simulink model "controller13"  (R2023a)
settings: Solver=FixedStepAuto  StartTime=0.0  StopTime=mdl.exe_time  RelTol=1e-3
values from neighbouring files (symbols this model uses):
  ctr2 = ctr    [s1_setup.m]    (also in step1_setup.m)
  lut = gen_lut    [s1_setup.m]    (also in thrust2voltage_lut_20230809.mat = ; thrust2voltage_lut_20230829.mat = )
  mdl = make_model(mdl,rsim)    [s1_setup.m]    (also in setup_controller_with_functions.m = make_model(flight_time); step1_setup.m)
  use_simulation = 1    [step1_setup_v1.m]
undefined symbols (not defined in the file or in its folder): Angle, Axis, DiscIntNeverNeededParam, rjsim, servo_config, Standard_Devices, UDP_Protocol
libraries: simulink x25, sldrtlib x9, robotcorelib x8, dspmathops x3, dspswit3 x2, shared6dofsys x2, dspfdesign x2, sharedtransform x1, sharedutil x1, matrix_library x1, shared6dof x1, simulink_extras x1
(part 2 of 3)

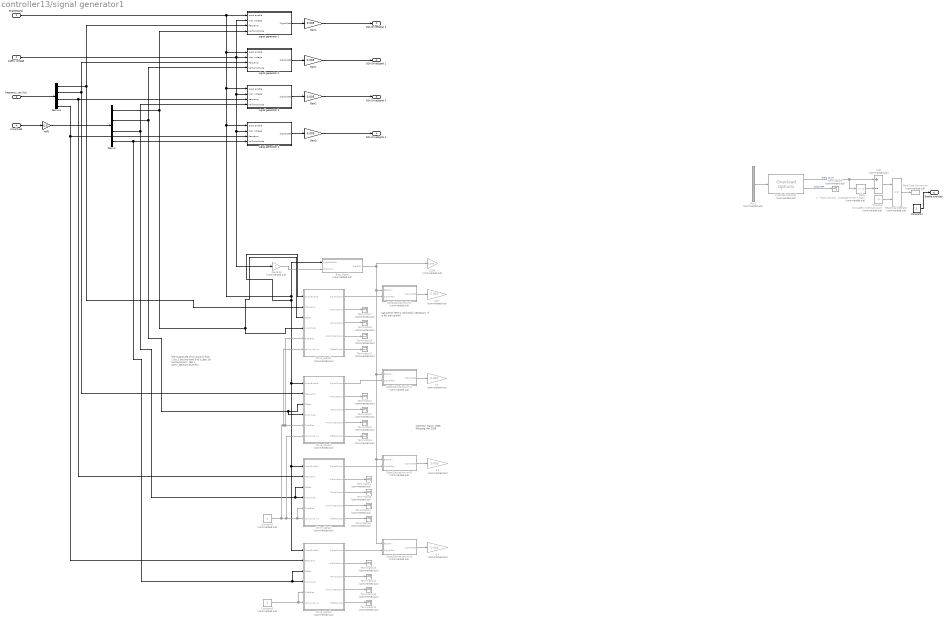
== system controller13/signal generator1 ==
  note: The magnitude of sin wave is from -1 to 1, but we want 0 to V_des. So we have 0.5*V_des + 0.5*V_des*sin(2*pi*f*t).
  note: Katie Byl
      | March, 2009
      |
      | Pakpong
      | Nov 2018
  note: saturation here is not totally necessary.
      | it is for pre-caution
  EnableSignal : Inport
  safety voltage : Inport  Port=2
  frequency_vec (hz) : Inport  Port=3
  Amplitude : Inport  Port=4
  0.2 : Gain  Commented=on  Gain=0.005
  0.3 : Gain  Commented=on  Gain=0.005
  0.4 : Gain  Commented=on  Gain=0.005
  1/200 : Gain  Commented=on  Gain=0.005
  Add : Sum  Commented=on  Inputs=+-
  Bias_Signal : Subsystem  Commented=on
  Constant : Constant  Commented=on  Value=ctr2.safety.overload.count
  Constant1 : Constant
  Constant2 : Constant  Commented=on  Value=0
  Constant3 : Constant  Commented=on  Value=0
  Data Type Conversion : DataTypeConversion  Commented=on  SaturateOnIntegerOverflow=off  RndMeth=Floor
  Delay : Delay  Commented=on  DelayLength=floor(ctr2.safety.overload.T*mdl.T_high)  InitialCondition=0
  Demux : Demux
  Demux1 : Demux
  Drive_Signal1 : Subsystem  Commented=on
  Drive_Signal2 : Subsystem  Commented=on
  Drive_Signal3 : Subsystem  Commented=on
  Drive_Signal4 : Subsystem  Commented=on
  Gain : Gain  Commented=on  Gain=0.005
  Gain{1..4} (4 alike) : Gain  Gain=0.005
  GainBias : Gain  Commented=on
  Mux2 : Mux  Commented=on
  Overload Options1 : slrealtimetgmanagement/Overload Options  Commented=on  startupDur=10  startupDurSrc=Tunable Parameter  maxOverload=1000  maxOverloadSrc=Tunable Parameter  TETFlag=on
  Relational Operator : RelationalOperator  Commented=on  Operator=<=  OutDataTypeStr=boolean  RndMeth=Simplest  InputSameDT=off
  SignalSaturationLimit : Subsystem  Commented=on
  SignalSaturationLimit1 : Subsystem  Commented=on
  SignalSaturationLimit2 : Subsystem  Commented=on
  SignalSaturationLimit3 : Subsystem  Commented=on
  Terminator{1..17} (17 alike) : Terminator  Commented=on
  half1 : Gain  Gain=0.5
  signal generator 1 : Subsystem
  signal generator 2 : Subsystem
  signal generator 3 : Subsystem
  signal generator 4 : Subsystem
  D2A DriveSignal 1 : Outport
  D2A DriveSignal 2 : Outport  Port=2
  D2A DriveSignal 3 : Outport  Port=3
  D2A DriveSignal 4 : Outport  Port=4
  Enable overload : Outport  Port=5
  wires:
  Bias_Signal/1(BiasD2A) -> 1/200/1, SignalSaturationLimit3/1(BiasMax), SignalSaturationLimit2/1(BiasMax), SignalSaturationLimit1/1(BiasMax), SignalSaturationLimit/1(BiasMax)
  EnableSignal/1 -> Drive_Signal1/1(QuasiEnable), Drive_Signal3/1(QuasiEnable), Drive_Signal2/1(QuasiEnable), Drive_Signal4/1(QuasiEnable), Bias_Signal/1(QuasiEnable), signal generator 4/1(quasi enable), signal generator 3/1(quasi enable), signal generator 2/1(quasi enable), signal generator 1/1(quasi enable)
  SignalSaturationLimit/1(SignalSatd) -> Gain/1
  GainBias/1 -> Bias_Signal/2(BiasVolts)
  SignalSaturationLimit1/1(SignalSatd) -> 0.2/1
  Amplitude/1 -> half1/1
  Drive_Signal3/4(AmplitudeOutput) -> Terminator15/1
  Drive_Signal3/2(WithoutRamp) -> Terminator13/1
  Drive_Signal3/3(RampOutput) -> Terminator14/1
  Drive_Signal3/5(OffsetOutput) -> Terminator12/1
  Drive_Signal2/3(RampOutput) -> Terminator8/1
  Drive_Signal2/4(AmplitudeOutput) -> Terminator11/1
  Drive_Signal3/1(SignalOutput) -> SignalSaturationLimit3/2(SignalRaw)
  Drive_Signal2/5(OffsetOutput) -> Terminator10/1
  Drive_Signal2/2(WithoutRamp) -> Terminator4/1
  Demux/3 -> Drive_Signal2/4(Amplitude), Drive_Signal2/3(Offset), signal generator 3/4(half amplitude)
  Demux/4 -> Drive_Signal3/4(Amplitude), Drive_Signal3/3(Offset), signal generator 4/4(half amplitude)
  Constant2/1 -> Drive_Signal1/6(split cycle mu), Drive_Signal1/5(PitchBias), Drive_Signal4/5(PitchBias), Drive_Signal4/6(split cycle mu), Drive_Signal2/5(PitchBias), Drive_Signal2/6(split cycle mu)
  Constant3/1 -> Drive_Signal3/5(PitchBias), Drive_Signal3/6(split cycle mu)
  SignalSaturationLimit2/1(SignalSatd) -> 0.3/1
  SignalSaturationLimit3/1(SignalSatd) -> 0.4/1
  Drive_Signal2/1(SignalOutput) -> SignalSaturationLimit2/2(SignalRaw)
  half1/1 -> Demux/1
  frequency_vec (hz)/1 -> Demux1/1
  Demux1/1 -> signal generator 1/3(frequency), Drive_Signal1/2(Frequency)
  Demux1/2 -> Drive_Signal4/2(Frequency), signal generator 2/3(frequency)
  Demux1/3 -> Drive_Signal2/2(Frequency), signal generator 3/3(frequency)
  Demux1/4 -> Drive_Signal3/2(Frequency), signal generator 4/3(frequency)
  Overload Options1/1 -> Delay/1, Add/1  "DrSig count"
  Overload Options1/2 -> Terminator3/1  "DrSig TET"
  Mux2/1 -> Overload Options1/1
  Delay/1 -> Add/2
  Add/1 -> Relational Operator/1
  Constant/1 -> Relational Operator/2
  Relational Operator/1 -> Data Type Conversion/1
  Drive_Signal4/1(SignalOutput) -> SignalSaturationLimit1/2(SignalRaw)
  Drive_Signal4/2(WithoutRamp) -> Terminator1/1
  Drive_Signal4/3(RampOutput) -> Terminator2/1
  Drive_Signal4/4(AmplitudeOutput) -> Terminator5/1
  Drive_Signal4/5(OffsetOutput) -> Terminator6/1
  Drive_Signal1/4(AmplitudeOutput) -> Terminator16/1
  Drive_Signal1/1(SignalOutput) -> SignalSaturationLimit/2(SignalRaw)
  Drive_Signal1/2(WithoutRamp) -> Terminator7/1
  Drive_Signal1/5(OffsetOutput) -> Terminator17/1
  Drive_Signal1/3(RampOutput) -> Terminator9/1
  Demux/1 -> Drive_Signal1/3(Offset), Drive_Signal1/4(Amplitude), signal generator 1/4(half amplitude)
  Constant1/1 -> Enable overload/1
  Demux/2 -> Drive_Signal4/4(Amplitude), Drive_Signal4/3(Offset), signal generator 2/4(half amplitude)
  safety voltage/1 -> GainBias/1, signal generator 4/2(max voltage), signal generator 3/2(max voltage), signal generator 1/2(max voltage), signal generator 2/2(max voltage)
  signal generator 2/1(SignalSatd) -> Gain1/1
  signal generator 3/1(SignalSatd) -> Gain2/1
  signal generator 4/1(SignalSatd) -> Gain3/1
  signal generator 1/1(SignalSatd) -> Gain4/1
  Gain3/1 -> D2A DriveSignal 4/1
  Gain2/1 -> D2A DriveSignal 3/1
  Gain1/1 -> D2A DriveSignal 2/1
  Gain4/1 -> D2A DriveSignal 1/1

== system controller13/signal safety (no imag & NaN) ==
  In1 : Inport
  Complex to Real-Imag{,1..3} (4 alike) : ComplexToRealImag
  Constant{,1..3} (4 alike) : Constant  Value=0
  Demux : Demux
  IsNaN{,1..3} (4 alike) : RelationalOperator  Operator=isNaN  OutDataTypeStr=boolean  RndMeth=Simplest  InputSameDT=off
  Mux : Mux
  Switch{1..3,17} (4 alike) : Switch  Criteria=u2 > Threshold  SaturateOnIntegerOverflow=off  InputSameDT=off
  Terminator{,1..3} (4 alike) : Terminator
  Output : Outport
  wires:
  In1/1 -> Demux/1
  IsNaN/1 -> Switch17/2
  Constant/1 -> Switch17/1
  Switch17/1 -> Complex to Real-Imag/1
  Complex to Real-Imag/2 -> Terminator/1
  Demux/1 -> Switch17/3, IsNaN/1
  Complex to Real-Imag1/2 -> Terminator1/1
  Complex to Real-Imag1/1 -> Mux/2
  IsNaN1/1 -> Switch1/2
  Switch1/1 -> Complex to Real-Imag1/1
  Demux/2 -> Switch1/3, IsNaN1/1
  Constant1/1 -> Switch1/1
  Complex to Real-Imag2/2 -> Terminator2/1
  Complex to Real-Imag2/1 -> Mux/3
  IsNaN2/1 -> Switch2/2
  Switch2/1 -> Complex to Real-Imag2/1
  Demux/3 -> Switch2/3, IsNaN2/1
  Constant2/1 -> Switch2/1
  Complex to Real-Imag3/2 -> Terminator3/1
  Complex to Real-Imag3/1 -> Mux/4
  IsNaN3/1 -> Switch3/2
  Demux/4 -> IsNaN3/1, Switch3/3
  Switch3/1 -> Complex to Real-Imag3/1
  Constant3/1 -> Switch3/1
  Mux/1 -> Output/1
  Complex to Real-Imag/1 -> Mux/1

== system controller13/stance climbing subsystem ==
  Action Port : ActionPort  ActionPortLabel=default:
  Constant7 : Constant  Value=[0;0;1]
  Out1 : Outport
  wires:
  Constant7/1 -> Out1/1

== system controller13/sync with Speedgoat ==
  Gain3 : Gain  OutDataTypeStr=uint8
  Packet Output2 : sldrtlib/Packet Output  SampleTime=1/2000  MaxMissedTicks=100  ShowMissedTicks=off  YieldWhenWaiting=off  DrvName=Standard_Devices/UDP_Protocol  DrvAddress=16300  DrvOptions=[0 24000 49 54 57 46 50 53 52 46 49 48 51 46 52 48 0 0 0 0 0 0 0 0 0 0 0 0 0 0 0 0 0 0 0 0 0 0 0 0 0 0 0 0 0 0 0 0 0 0 0 0 0 0 0 0 0 0 0 0 0 0 0 0 0 0 0 0 0 0 0 0 0 0 0 0 0 0 0 0 0 0 0 0 0 0 0 0 0 0 0 0 0 0 0 0 0 0 0 0 0 0 0 0 0 0 0 0 0 0 0 0 0 0 0 0 0 0 0 0 0 0 0 0 0 0 0 0 0 0 0 0 0 0 0 0 0 0 0 0 0 0 0 0 0 0 0 0 0 0 0 0 0 0 0 0 0 0 0 0 0 0 0 0 0 0 0 0 0 0 0 0 0 0 0 0 0 0 0 0 0 0 0 0 0 0 0 0 0 0 0 0 0 0 0 0 0 0 0 0 0 0 0 0 0 0 0 0 0 0 0 0 0 0 0 0 0 0 0 0 0 0 0 0 0 0 0 0 0 0 0 0 0 0 0 0 0 0 0 0 0 0 0 0 0 0 0 0 0 0 0 0 0 0 0 0]  PacketSize=1  DataTypes='1*uint8'  ShowReady=off  ShowError=off  PacketID=1  ByteOrder=1  InitialValue=[]  FinalValue=[]
      settings: AttributesFormatString=UDP Protocol [16300]
  Pulse Generator : DiscretePulseGenerator  Period=1000  PulseWidth=500  SampleTime=1/2000
  Scope : Scope
  wires:
  Pulse Generator/1 -> Gain3/1
  Gain3/1 -> Packet Output2/1, Scope/1

== system controller13/voltage safety (no imag & NaN) ==
  In1 : Inport
  Complex to Real-Imag{,1..3} (4 alike) : ComplexToRealImag
  Delay{,1..3} (4 alike) : Delay  DelayLength=1
  Demux : Demux
  IsNaN{,1..3} (4 alike) : RelationalOperator  Operator=isNaN  OutDataTypeStr=boolean  RndMeth=Simplest  InputSameDT=off
  Mux : Mux
  Switch{1..3,17} (4 alike) : Switch  Criteria=u2 > Threshold  SaturateOnIntegerOverflow=off  InputSameDT=off
  Terminator{,1..3} (4 alike) : Terminator
  Output : Outport
  wires:
  In1/1 -> Demux/1
  IsNaN/1 -> Switch17/2
  Switch17/1 -> Delay1/1, Complex to Real-Imag/1
  Complex to Real-Imag/2 -> Terminator/1
  Demux/1 -> Switch17/3, IsNaN/1
  Complex to Real-Imag1/2 -> Terminator1/1
  Complex to Real-Imag1/1 -> Mux/2
  IsNaN1/1 -> Switch1/2
  Switch1/1 -> Delay/1, Complex to Real-Imag1/1
  Demux/2 -> Switch1/3, IsNaN1/1
  Complex to Real-Imag2/2 -> Terminator2/1
  Complex to Real-Imag2/1 -> Mux/3
  IsNaN2/1 -> Switch2/2
  Switch2/1 -> Delay2/1, Complex to Real-Imag2/1
  Demux/3 -> Switch2/3, IsNaN2/1
  Complex to Real-Imag3/2 -> Terminator3/1
  Complex to Real-Imag3/1 -> Mux/4
  IsNaN3/1 -> Switch3/2
  Demux/4 -> IsNaN3/1, Switch3/3
  Switch3/1 -> Delay3/1, Complex to Real-Imag3/1
  Mux/1 -> Output/1
  Complex to Real-Imag/1 -> Mux/1
  Delay/1 -> Switch1/1
  Delay1/1 -> Switch17/1
  Delay2/1 -> Switch2/1
  Delay3/1 -> Switch3/1

== system controller13/yaw-free attitude controller ==
  desired_z_b : Inport
  R : Inport  Port=2
  omega_b : Inport  Port=3
  Add1 : Sum  Inputs=-+|
  Constant4 : Constant  Value=[0;0;1]
  Cross Product : vrlib/Utilities/Cross Product
  Gain : Gain  Gain=-1
  Matrix Multiply2 : Product  Multiplication=Matrix(*)
  Matrix Multiply5 : Product  Multiplication=Matrix(*)
  Product1 : Product
  Product2 : Product
  Transpose : Math  Operator=transpose
  d_gain : Constant  Value=[30;37;0]
  p_gain : Constant  Value=[350;600;0]
  z_b : Outport
  torque_b : Outport  Port=2
  wires:
  d_gain/1 -> Product1/2
  desired_z_b/1 -> Cross Product/1
  Constant4/1 -> Matrix Multiply2/2
  Matrix Multiply2/1 -> z_b/1, Cross Product/2
  R/1 -> Matrix Multiply2/1, Transpose/1
  Gain/1 -> Matrix Multiply5/2
  Cross Product/1 -> Gain/1
  Product1/1 -> Add1/1
  Add1/1 -> torque_b/1
  omega_b/1 -> Product1/1
  Transpose/1 -> Matrix Multiply5/1  "R^T"
  Matrix Multiply5/1 -> Product2/1
  p_gain/1 -> Product2/2
  Product2/1 -> Add1/2

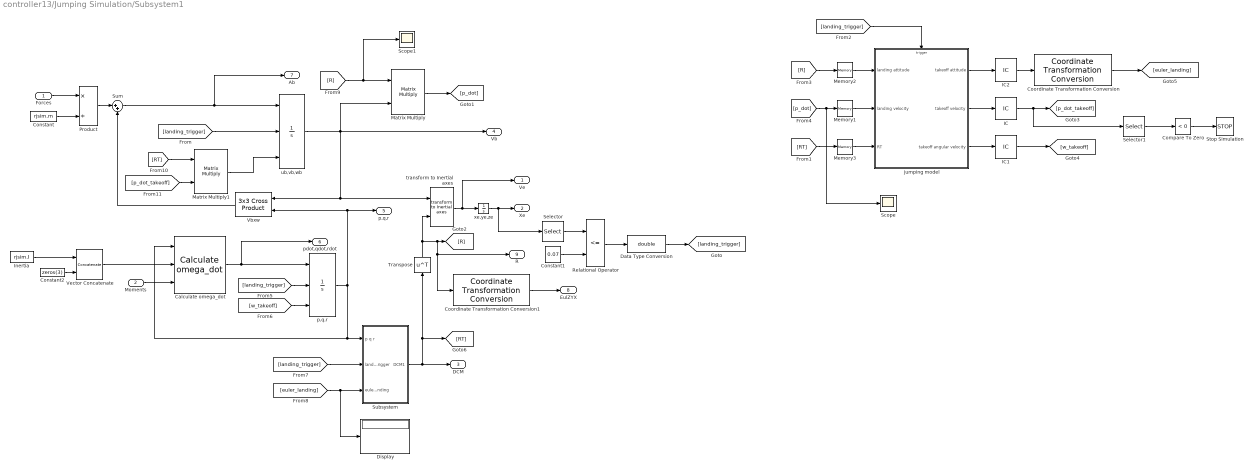
== system controller13/Jumping Simulation/Subsystem1 ==
  Forces : Inport  OutDataTypeStr=double  Unit=N  PortDimensions=3
  Moments : Inport  Port=2  OutDataTypeStr=double  Unit=N*m  PortDimensions=3
  Calculate omega_dot : shared6dofsys/Calculate omega_dot  aMode=aMode
  Compare To Zero : simulink/Logic and Bit Operations/Compare To Zero  relop=<  OutDataTypeStr=boolean
  Constant : Constant  Value=rjsim.m  OutDataTypeStr=Inherit: Inherit via back propagation
  Constant1 : Constant  Value=0.07
  Constant2 : Constant  Value=zeros(3)
  Coordinate Transformation Conversion : robotcorelib/Coordinate Transformation Conversion  InputRepresentation=Rotation Matrix  InputEulerSequence=ZYX  ShowTrVecInputPort=on  OutputRepresentation=Euler Angles  OutputEulerSequence=ZYX  ShowTrVecOutputPort=on  SimulateUsing=Interpreted execution
      settings: LibrarySourceBlock=navlib/Utilities/Coordinate Transformation Conversion
  Coordinate Transformation Conversion1 : robotcorelib/Coordinate Transformation Conversion  InputRepresentation=Rotation Matrix  InputEulerSequence=ZYX  ShowTrVecInputPort=on  OutputRepresentation=Euler Angles  OutputEulerSequence=ZYX  ShowTrVecOutputPort=on  SimulateUsing=Interpreted execution
      settings: LibrarySourceBlock=navlib/Utilities/Coordinate Transformation Conversion
  Data Type Conversion : DataTypeConversion  OutDataTypeStr=double  SaturateOnIntegerOverflow=off  RndMeth=Floor
  Display : Display
  IC : InitialCondition  Value=rjsim.v0
  IC1 : InitialCondition  Value=[0,0,0]
  IC2 : InitialCondition  Value=rjsim.rotm0
  Inertia : Constant  Value=rjsim.I  OutDataTypeStr=Inherit: Inherit via back propagation
  Matrix Multiply : Product  Multiplication=Matrix(*)
  Matrix Multiply1 : Product  Multiplication=Matrix(*)
  Memory1 : Memory
  Memory2 : Memory
  Memory3 : Memory
  Product : Product  Inputs=*/  SaturateOnIntegerOverflow=on  OutDataTypeStr=Inherit: Same as first input
  Relational Operator : RelationalOperator  Operator=<=  OutDataTypeStr=boolean  RndMeth=Simplest  InputSameDT=off
  Scope : Scope
  Scope1 : Scope
  Selector : Selector  InputPortWidth=3  IndexOptions=Index vector (dialog)  Indices=[3]  OutputSizes=1
  Selector1 : Selector  InputPortWidth=3  IndexOptions=Index vector (dialog)  Indices=[3]  OutputSizes=1
  Stop Simulation : Stop
  Subsystem : Subsystem
  Sum : Sum  Inputs=|++  SaturateOnIntegerOverflow=on
  Transpose : Math  Operator=transpose  SignedPower=on
  Vbxw : sharedutil/3x3 Cross Product  aMode=aMode
  Vector Concatenate : Concatenate  Mode=Multidimensional array
  jumping model : Subsystem  TreatAsAtomicUnit=on
  "p,q,r " : Integrator  ExternalReset=rising  InitialConditionSource=external  InitialCondition=[0,0,0]
  "transform to Inertial axes " : shared6dof/6DOF (Euler Angles)/transform to Inertial axes   SystemSampleTime=-1  VariantActivationTime=update diagram  Latency=0  AutoFrameSizeCalculation=off
  ub,vb,wb : Integrator  ExternalReset=rising  InitialConditionSource=external  InitialCondition=[0,0,0]
  xe,ye,ze : Integrator  InitialCondition=rjsim.p0
  Ve : Outport  OutDataTypeStr=double  Unit=m/s  VectorParamsAs1DForOutWhenUnconnected=off
  Xe : Outport  Port=2  OutDataTypeStr=double  Unit=m  VectorParamsAs1DForOutWhenUnconnected=off
  DCM : Outport  Port=3  OutDataTypeStr=double  Unit=1  VectorParamsAs1DForOutWhenUnconnected=off
  Vb : Outport  Port=4  OutDataTypeStr=double  Unit=m/s  VectorParamsAs1DForOutWhenUnconnected=off
  p,q,r : Outport  Port=5  OutDataTypeStr=double  Unit=rad/s  VectorParamsAs1DForOutWhenUnconnected=off
  pdot,qdot,rdot : Outport  Port=6  OutDataTypeStr=double  Unit=rad/s^2  VectorParamsAs1DForOutWhenUnconnected=off
  Ab : Outport  Port=7  OutDataTypeStr=double  Unit=m/s^2  VectorParamsAs1DForOutWhenUnconnected=off
  EulZYX : Outport  Port=8
  R : Outport  Port=9
  wires:
  "transform to Inertial axes "/1 -> Ve/1, xe,ye,ze/1
  Constant/1 -> Product/2
  Product/1 -> Sum/1
  xe,ye,ze/1 -> Selector/1, Xe/1
  ub,vb,wb/1 -> Vb/1, Matrix Multiply/2, Vbxw/1, "transform to Inertial axes "/1
  Sum/1 -> Ab/1, ub,vb,wb/1
  Vbxw/1 -> Sum/2
  "p,q,r "/1 -> Calculate omega_dot/1, Subsystem/1("p q r "), Vbxw/2, p,q,r/1
  Subsystem/1(DCM1) -> Transpose/1, [RT], DCM/1
  Forces/1 -> Product/1
  Transpose/1 -> Coordinate Transformation Conversion1/1, R/1, [R], "transform to Inertial axes "/2
  Calculate omega_dot/1 -> pdot,qdot,rdot/1, "p,q,r "/1
  Moments/1 -> Calculate omega_dot/3
  Vector Concatenate/1 -> Calculate omega_dot/2
  Constant2/1 -> Vector Concatenate/2
  Inertia/1 -> Vector Concatenate/1
  Constant1/1 -> Relational Operator/2
  Selector/1 -> Relational Operator/1
  Relational Operator/1 -> Data Type Conversion/1
  [landing_trigger] -> ub,vb,wb/2
  [landing_trigger] -> jumping model/Trigger
  [R] -> Memory2/1
  [p_dot] -> Scope/1, Memory1/1
  Memory1/1 -> jumping model/2(landing velocity)
  Memory2/1 -> jumping model/1(landing attitude)
  jumping model/2(takeoff velocity) -> IC/1
  [landing_trigger] -> "p,q,r "/2
  jumping model/3(takeoff angular velocity) -> IC1/1
  [w_takeoff] -> "p,q,r "/3
  [landing_trigger] -> Subsystem/2(landing trigger)
  jumping model/1(takeoff attitude) -> IC2/1
  Coordinate Transformation Conversion/1 -> [euler_landing]
  Data Type Conversion/1 -> [landing_trigger]
  IC/1 -> Selector1/1, [p_dot_takeoff]
  IC1/1 -> [w_takeoff]
  IC2/1 -> Coordinate Transformation Conversion/1
  [R] -> Scope1/1, Matrix Multiply/1
  Matrix Multiply/1 -> [p_dot]
  [RT] -> Matrix Multiply1/1
  [p_dot_takeoff] -> Matrix Multiply1/2
  Matrix Multiply1/1 -> ub,vb,wb/3
  Coordinate Transformation Conversion1/1 -> EulZYX/1
  [RT] -> Memory3/1
  Memory3/1 -> jumping model/3(RT)
  Selector1/1 -> Compare To Zero/1
  Compare To Zero/1 -> Stop Simulation/1
  [euler_landing] -> Display/1, Subsystem/3(euler_landing)

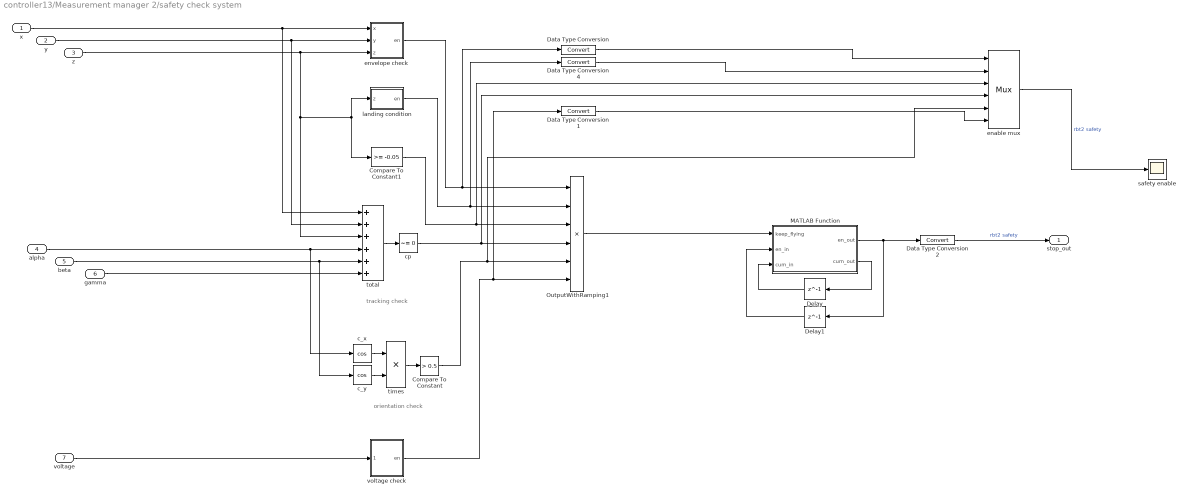
== system controller13/Measurement manager 2/safety check system ==
  note: orientation check
  note: tracking check
  x : Inport
  y : Inport  Port=2
  z : Inport  Port=3
  alpha : Inport  Port=4
  beta : Inport  Port=5
  gamma : Inport  Port=6
  voltage : Inport  Port=7
  Compare To Constant : simulink/Logic and Bit Operations/Compare To Constant  relop=>  const=0.5  OutDataTypeStr=uint8
  Compare To Constant1 : simulink/Logic and Bit Operations/Compare To Constant  relop=>=  const=-0.05  OutDataTypeStr=uint8
  Data Type Conversion{,1..2,4} (4 alike) : DataTypeConversion  SaturateOnIntegerOverflow=off  RndMeth=Floor
  Delay : Delay  DelayLength=1
  Delay1 : Delay  DelayLength=1  InitialCondition=1
  MATLAB Function : MATLAB Function  TreatAsAtomicUnit=on
  OutputWithRamping1 : Product  Inputs=6  RndMeth=Zero
  c_x : Trigonometry  Operator=cos
  c_y : Trigonometry  Operator=cos
  cp : simulink/Logic and Bit Operations/Compare To Zero  relop=~=  OutDataTypeStr=uint8
  enable mux : Mux  Inputs=6
      settings: DisplayOption=signals
  envelope check : MATLAB Function  TreatAsAtomicUnit=on
  landing condition : Subsystem
  safety enable : Scope
  times : Product  RndMeth=Zero
  total : Sum  Inputs=++++++
  voltage check : MATLAB Function  TreatAsAtomicUnit=on  SystemSampleTime=mdl.T
  stop_out : Outport
  wires:
  Compare To Constant1/1 -> enable mux/3, OutputWithRamping1/3
  y/1 -> envelope check/2(y), total/2
  cp/1 -> enable mux/4, OutputWithRamping1/4
  envelope check/1(en) -> Data Type Conversion/1, OutputWithRamping1/1
  enable mux/1 -> safety enable/1  "rbt2 safety"
  landing condition/1(en) -> Data Type Conversion4/1, OutputWithRamping1/2
  Data Type Conversion/1 -> enable mux/1
  times/1 -> Compare To Constant/1
  voltage check/1(en) -> Data Type Conversion1/1, OutputWithRamping1/6
  z/1 -> total/3, Compare To Constant1/1, landing condition/1(z), envelope check/3(z)
  Compare To Constant/1 -> enable mux/5, OutputWithRamping1/5
  total/1 -> cp/1
  Data Type Conversion4/1 -> enable mux/2
  x/1 -> total/1, envelope check/1(x)
  alpha/1 -> total/4, c_x/1
  beta/1 -> total/5, c_y/1
  c_x/1 -> times/1
  c_y/1 -> times/2
  Data Type Conversion1/1 -> enable mux/6
  voltage/1 -> voltage check/1(voltage)
  gamma/1 -> total/6
  OutputWithRamping1/1 -> MATLAB Function/1(keep_flying)
  Delay1/1 -> MATLAB Function/2(en_in)
  MATLAB Function/1(en_out) -> Delay1/1, Data Type Conversion2/1
  Delay/1 -> MATLAB Function/3(cum_in)
  MATLAB Function/2(cum_out) -> Delay/1
  Data Type Conversion2/1 -> stop_out/1  "rbt2 safety"

== system controller13/Subsystem6/Subsystem4 ==
  In1 : Inport
  data ready : Inport  Port=2
  Add1 : Sum  Inputs=+-
  Add2 : Sum  Inputs=+-
  Digital Clock : DigitalClock  SampleTime=1/10000
  If : If  IfExpression=u1 == 0
  If Action Subsystem : Subsystem  TreatAsAtomicUnit=on
  If Action Subsystem1 : Subsystem  TreatAsAtomicUnit=on
  Merge : Merge
  Triggered Subsystem : Subsystem  TreatAsAtomicUnit=on
  p dot : Outport
  wires:
  In1/1 -> Triggered Subsystem/1(In1)
  data ready/1 -> Triggered Subsystem/Trigger
  Triggered Subsystem/1(Out1) -> Add1/1
  Triggered Subsystem/2(Output) -> Add1/2
  Triggered Subsystem/3(Output1) -> Add2/1
  Triggered Subsystem/4(Output2) -> Add2/2
  Add1/1 -> If Action Subsystem/1(In1)
  Add2/1 -> If Action Subsystem/2(In2), If/1
  If/2 -> If Action Subsystem/Action
  If/1 -> If Action Subsystem1/Action
  If Action Subsystem1/1(Out1) -> Merge/2
  If Action Subsystem/1(Out1) -> Merge/1
  Merge/1 -> p dot/1
  Digital Clock/1 -> Triggered Subsystem/2(In2)

== system controller13/Subsystem6/Subsystem5 ==
  euler_angles : Inport
  data ready : Inport  Port=2
  sim enable : Inport  Port=3
  Add1 : Sum  Inputs=+-
  Add2 : Sum  Inputs=+-
  Add3 : Sum  Inputs=+-
  Delay : Delay  DelayLength=25  InitialCondition=zeros(9,25)
  Digital Clock : DigitalClock  SampleTime=1/10000
  Gain : Gain  Gain=1/(25/10000)
  If : If  IfExpression=u1 == 0
  If Action Subsystem : Subsystem  TreatAsAtomicUnit=on
  If Action Subsystem1 : Subsystem  TreatAsAtomicUnit=on
  Merge : Merge
  Rotation Matrix : MATLAB Function  TreatAsAtomicUnit=on
  Rotation Matrix1 : MATLAB Function  TreatAsAtomicUnit=on
  Switch1 : Switch  Criteria=u2 > Threshold  SaturateOnIntegerOverflow=off  InputSameDT=off
  Triggered Subsystem : Subsystem  TreatAsAtomicUnit=on
  R : Outport
  Rdot : Outport  Port=2
  Omega : Outport  Port=3
  wires:
  Triggered Subsystem/1(Out1) -> Add1/1
  Triggered Subsystem/3(Output1) -> Add2/1
  Triggered Subsystem/4(Output2) -> Add2/2
  If Action Subsystem1/1(Out1) -> Merge/2
  If Action Subsystem/1(Out1) -> Merge/1
  Triggered Subsystem/2(Output) -> Add1/2
  Digital Clock/1 -> Triggered Subsystem/2(In2)
  data ready/1 -> Triggered Subsystem/Trigger
  Add2/1 -> If Action Subsystem/2(In2), If/1
  If/2 -> If Action Subsystem/Action
  If/1 -> If Action Subsystem1/Action
  Add1/1 -> If Action Subsystem/1(In1)
  euler_angles/1 -> Rotation Matrix/1(euler_angles)
  Rotation Matrix/1(R) -> Triggered Subsystem/1(R), Delay/1, Add3/1, R/1, Rotation Matrix1/1(R)
  Rotation Matrix1/1(w) -> Omega/1  "p_filt"
  Delay/1 -> Add3/2
  Add3/1 -> Gain/1
  Gain/1 -> Switch1/1
  sim enable/1 -> Switch1/2
  Merge/1 -> Switch1/3
  Switch1/1 -> Rotation Matrix1/2(Rdot), Rdot/1  "p_raw"

== system controller13/UDP send to Arduino/HV amplifier gains ==
  high voltage 1 : Inport
  high voltage 2 : Inport  Port=2
  high voltage 3 : Inport  Port=3
  high voltage 4 : Inport  Port=4
  Gain{4..7} (4 alike) : Gain
  DAC voltage 1 : Outport
  DAC voltage 2 : Outport  Port=2
  DAC voltage 3 : Outport  Port=3
  DAC voltage 4 : Outport  Port=4
  wires:
  Gain5/1 -> DAC voltage 2/1  "DAC voltage 2"
  Gain4/1 -> DAC voltage 1/1  "DAC voltage 1"
  high voltage 2/1 -> Gain5/1
  Gain7/1 -> DAC voltage 4/1  "DAC voltage 4"
  high voltage 1/1 -> Gain4/1
  Gain6/1 -> DAC voltage 3/1  "DAC voltage 3"
  high voltage 3/1 -> Gain6/1
  high voltage 4/1 -> Gain7/1

== system controller13/UDP send to Arduino/UDP send to Arduino DAC ==
  note: Aptinex DAC 20230818
  DAC1 : Inport
  DAC2 : Inport  Port=2
  DAC3 : Inport  Port=3
  DAC4 : Inport  Port=4
  DO2 : Inport  Port=5  OutDataTypeStr=boolean
  Bit Set : simulink/Logic and Bit Operations/Bit Set  iBit=12
  Demux : Demux
  Gain : Gain  Gain=4095/10.28  OutDataTypeStr=uint16
  Gain1 : Gain  Gain=4095/10.68  OutDataTypeStr=uint16
  Gain2 : Gain  Gain=4095/10.44  OutDataTypeStr=uint16
  Gain3 : Gain  Gain=4095/10  OutDataTypeStr=uint16
  Mux : Mux
  Mux1 : Mux
  Saturation : Saturate  UpperLimit=10  LowerLimit=0
  Switch : Switch  Criteria=u2 ~= 0  OutDataTypeStr=uint16  SaturateOnIntegerOverflow=off  InputSameDT=off
  Output : Outport
  wires:
  Gain3/1 -> Mux1/4  "UDP uint16 4"
  Gain1/1 -> Mux1/2  "UDP uint16 2"
  Gain/1 -> Bit Set/1, Switch/3  "UDP uint16 1"
  Gain2/1 -> Mux1/3  "UDP uint16 3"
  DO2/1 -> Switch/2
  Bit Set/1 -> Switch/1
  Mux1/1 -> Output/1
  Switch/1 -> Mux1/1
  Demux/1 -> Gain/1
  Demux/2 -> Gain1/1
  Demux/3 -> Gain2/1
  Demux/4 -> Gain3/1
  DAC1/1 -> Mux/1  "DAC voltage 1"
  DAC2/1 -> Mux/2  "DAC voltage 2"
  DAC3/1 -> Mux/3  "DAC voltage 3"
  DAC4/1 -> Mux/4  "DAC voltage 4"
  Mux/1 -> Saturation/1
  Saturation/1 -> Demux/1

== system controller13/get xy ini/Subsystem ==
  In1 : Inport
  Trigger : TriggerPort  VariantControl=Variant  PortDimensions=1
  Out1 : Outport
  wires:
  In1/1 -> Out1/1

== system controller13/servo control/servowrite ==
  In1 : Inport
  Add : Sum  Inputs=|+-
  Add1 : Sum  Inputs=|+-
  Add2 : Sum  Inputs=|+-
  Constant2 : Constant  Value=700
  Constant3 : Constant  Value=90
  Constant4 : Constant  Value=-1500
  Data Type Conversion : DataTypeConversion  OutDataTypeStr=uint16  SaturateOnIntegerOverflow=off  RndMeth=Floor
  Gain : Gain  Gain=800/76
  Packet Output : sldrtlib/Packet Output  SampleTime=1/400  MaxMissedTicks=100  ShowMissedTicks=off  YieldWhenWaiting=off  DrvName=Standard_Devices/UDP_Protocol  DrvAddress=25005  DrvOptions=[0 25000 49 54 57 46 50 53 52 46 49 48 51 46 52 57 0 0 0 0 0 0 0 0 0 0 0 0 0 0 0 0 0 0 0 0 0 0 0 0 0 0 0 0 0 0 0 0 0 0 0 0 0 0 0 0 0 0 0 0 0 0 0 0 0 0 0 0 0 0 0 0 0 0 0 0 0 0 0 0 0 0 0 0 0 0 0 0 0 0 0 0 0 0 0 0 0 0 0 0 0 0 0 0 0 0 0 0 0 0 0 0 0 0 0 0 0 0 0 0 0 0 0 0 0 0 0 0 0 0 0 0 0 0 0 0 0 0 0 0 0 0 0 0 0 0 0 0 0 0 0 0 0 0 0 0 0 0 0 0 0 0 0 0 0 0 0 0 0 0 0 0 0 0 0 0 0 0 0 0 0 0 0 0 0 0 0 0 0 0 0 0 0 0 0 0 0 0 0 0 0 0 0 0 0 0 0 0 0 0 0 0 0 0 0 0 0 0 0 0 0 0 0 0 0 0 0 0 0 0 0 0 0 0 0 0 0 0 0 0 0 0 0 0 0 0 0 0 0 0 0 0 0 0 0 0]  PacketSize=2  DataTypes='1*uint16'  ShowReady=off  ShowError=off  PacketID=1  ByteOrder=1  InitialValue=[]  FinalValue=[]
      settings: AttributesFormatString=UDP Protocol [25005]
  Saturation : Saturate  UpperLimit=2300  LowerLimit=700
  wires:
  Add2/1 -> Saturation/1
  Data Type Conversion/1 -> Packet Output/1
  Constant2/1 -> Add/2
  Constant4/1 -> Add2/2
  Gain/1 -> Add2/1
  Add/1 -> Data Type Conversion/1
  In1/1 -> Add1/1
  Saturation/1 -> Add/1
  Constant3/1 -> Add1/2
  Add1/1 -> Gain/1

== system controller13/signal generator1/Bias_Signal ==
  note: time constant = 0.002sec
  QuasiEnable : Inport
  BiasVolts : Inport  Port=2
  AveragedBias : Subsystem
  PreGain : Gain
  Product : Product  RndMeth=Zero
  SIgnalForRamp_binary : Subsystem
  SaturatingRamp : DiscreteIntegrator  gainval=100  SampleTime=-1  LimitOutput=on  UpperSaturationLimit=1  LowerSaturationLimit=0  ICPrevOutput=DiscIntNeverNeededParam  ICPrevScaledInput=DiscIntNeverNeededParam
  BiasD2A : Outport
  wires:
  PreGain/1 -> BiasD2A/1
  BiasVolts/1 -> AveragedBias/1(In1)
  QuasiEnable/1 -> SIgnalForRamp_binary/1(In1)
  SIgnalForRamp_binary/1(Out1) -> SaturatingRamp/1
  SaturatingRamp/1 -> Product/1
  AveragedBias/1(Out1) -> Product/2
  Product/1 -> PreGain/1

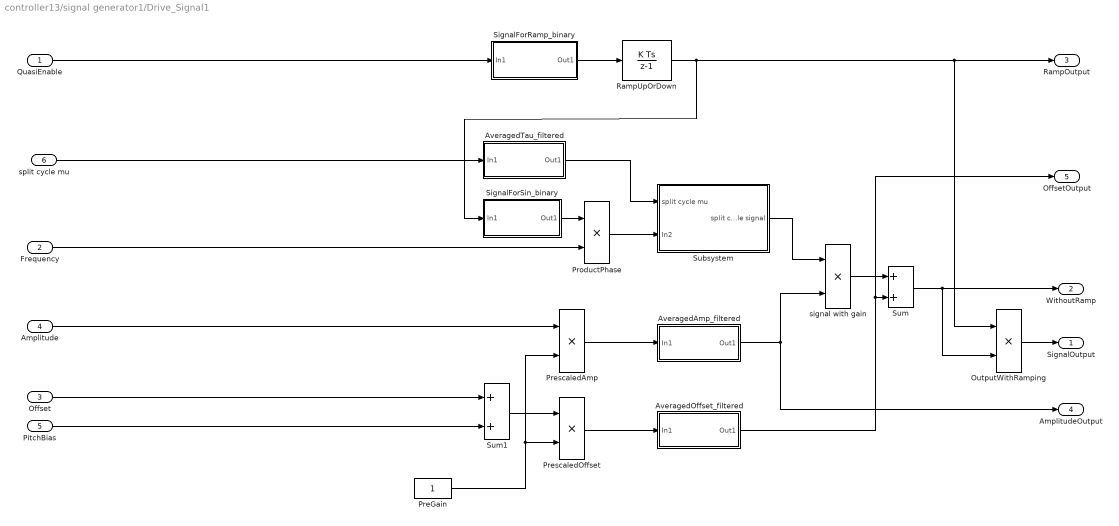
== system controller13/signal generator1/Drive_Signal1 ==
  QuasiEnable : Inport
  Frequency : Inport  Port=2
  Offset : Inport  Port=3
  Amplitude : Inport  Port=4
  PitchBias : Inport  Port=5
  split cycle mu : Inport  Port=6
  AveragedAmp_filtered : Subsystem
  AveragedOffset_filtered : Subsystem
  AveragedTau_filtered : Subsystem
  OutputWithRamping : Product  RndMeth=Zero
  PreGain : Constant
  PrescaledAmp : Product  RndMeth=Zero
  PrescaledOffset : Product  RndMeth=Zero
  ProductPhase : Product  RndMeth=Zero
  RampUpOrDown : DiscreteIntegrator  gainval=100  SampleTime=-1  LimitOutput=on  UpperSaturationLimit=1  LowerSaturationLimit=0  ICPrevOutput=DiscIntNeverNeededParam  ICPrevScaledInput=DiscIntNeverNeededParam
  SignalForRamp_binary : Subsystem
  SignalForSin_binary : Subsystem
  Subsystem : Subsystem
  Sum : Sum
  Sum1 : Sum
  signal with gain : Product  RndMeth=Zero
  SignalOutput : Outport
  WithoutRamp : Outport  Port=2
  RampOutput : Outport  Port=3
  AmplitudeOutput : Outport  Port=4
  OffsetOutput : Outport  Port=5
  wires:
  PrescaledAmp/1 -> AveragedAmp_filtered/1(In1)
  Sum/1 -> OutputWithRamping/2, WithoutRamp/1
  RampUpOrDown/1 -> RampOutput/1, OutputWithRamping/1, SignalForSin_binary/1(In1)
  QuasiEnable/1 -> SignalForRamp_binary/1(In1)
  SignalForRamp_binary/1(Out1) -> RampUpOrDown/1
  Amplitude/1 -> PrescaledAmp/1
  signal with gain/1 -> Sum/1
  Frequency/1 -> ProductPhase/2
  SignalForSin_binary/1(Out1) -> ProductPhase/1
  ProductPhase/1 -> Subsystem/2(In2)
  AveragedOffset_filtered/1(Out1) -> Sum/2, OffsetOutput/1
  PrescaledOffset/1 -> AveragedOffset_filtered/1(In1)
  PreGain/1 -> PrescaledAmp/2, PrescaledOffset/2
  OutputWithRamping/1 -> SignalOutput/1
  AveragedAmp_filtered/1(Out1) -> signal with gain/2, AmplitudeOutput/1
  Sum1/1 -> PrescaledOffset/1
  Offset/1 -> Sum1/1
  PitchBias/1 -> Sum1/2
  AveragedTau_filtered/1(Out1) -> Subsystem/1(split cycle mu)
  split cycle mu/1 -> AveragedTau_filtered/1(In1)
  Subsystem/1(split cycle signal) -> signal with gain/1

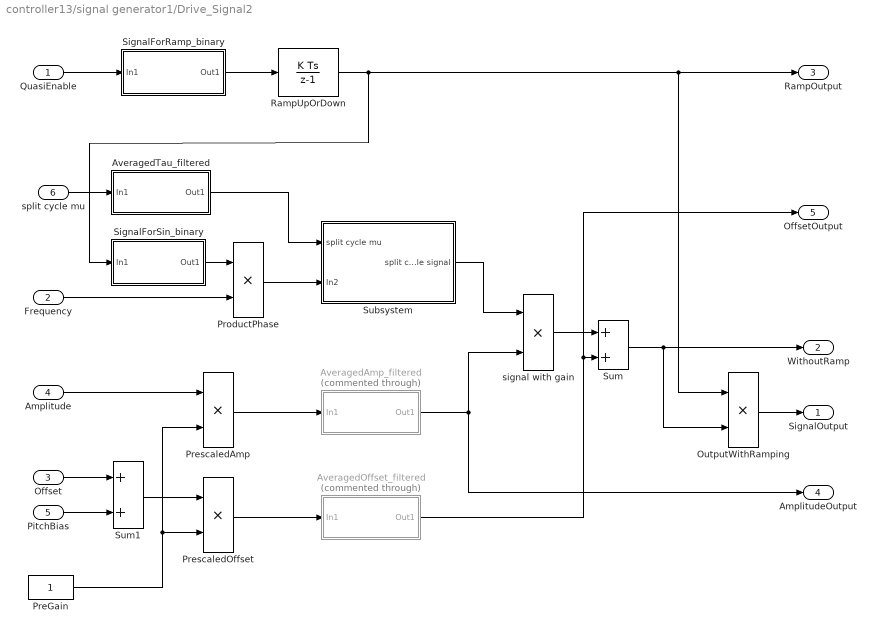
== system controller13/signal generator1/Drive_Signal2 ==
  QuasiEnable : Inport
  Frequency : Inport  Port=2
  Offset : Inport  Port=3
  Amplitude : Inport  Port=4
  PitchBias : Inport  Port=5
  split cycle mu : Inport  Port=6
  AveragedAmp_filtered : Subsystem  Commented=through
  AveragedOffset_filtered : Subsystem  Commented=through
  AveragedTau_filtered : Subsystem
  OutputWithRamping : Product  RndMeth=Zero
  PreGain : Constant
  PrescaledAmp : Product  RndMeth=Zero
  PrescaledOffset : Product  RndMeth=Zero
  ProductPhase : Product  RndMeth=Zero
  RampUpOrDown : DiscreteIntegrator  gainval=100  SampleTime=-1  LimitOutput=on  UpperSaturationLimit=1  LowerSaturationLimit=0  ICPrevOutput=DiscIntNeverNeededParam  ICPrevScaledInput=DiscIntNeverNeededParam
  SignalForRamp_binary : Subsystem
  SignalForSin_binary : Subsystem
  Subsystem : Subsystem
  Sum : Sum
  Sum1 : Sum
  signal with gain : Product  RndMeth=Zero
  SignalOutput : Outport
  WithoutRamp : Outport  Port=2
  RampOutput : Outport  Port=3
  AmplitudeOutput : Outport  Port=4
  OffsetOutput : Outport  Port=5
  wires:
  PrescaledAmp/1 -> AveragedAmp_filtered/1(In1)
  Sum/1 -> OutputWithRamping/2, WithoutRamp/1
  RampUpOrDown/1 -> RampOutput/1, OutputWithRamping/1, SignalForSin_binary/1(In1)
  QuasiEnable/1 -> SignalForRamp_binary/1(In1)
  SignalForRamp_binary/1(Out1) -> RampUpOrDown/1
  Amplitude/1 -> PrescaledAmp/1
  signal with gain/1 -> Sum/1
  Frequency/1 -> ProductPhase/2
  SignalForSin_binary/1(Out1) -> ProductPhase/1
  ProductPhase/1 -> Subsystem/2(In2)
  AveragedOffset_filtered/1(Out1) -> Sum/2, OffsetOutput/1
  PrescaledOffset/1 -> AveragedOffset_filtered/1(In1)
  PreGain/1 -> PrescaledAmp/2, PrescaledOffset/2
  OutputWithRamping/1 -> SignalOutput/1
  AveragedAmp_filtered/1(Out1) -> signal with gain/2, AmplitudeOutput/1
  Sum1/1 -> PrescaledOffset/1
  Offset/1 -> Sum1/1
  PitchBias/1 -> Sum1/2
  AveragedTau_filtered/1(Out1) -> Subsystem/1(split cycle mu)
  split cycle mu/1 -> AveragedTau_filtered/1(In1)
  Subsystem/1(split cycle signal) -> signal with gain/1

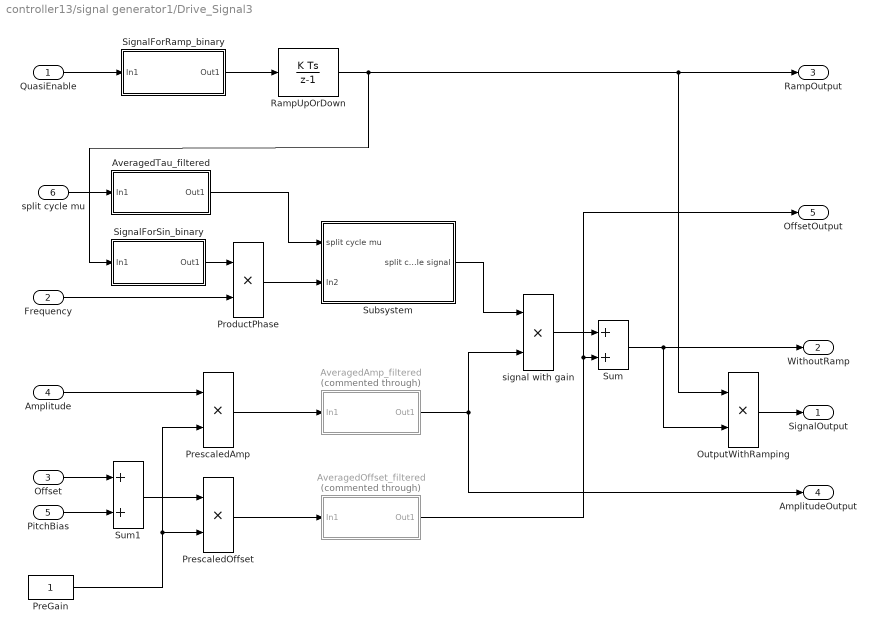
== system controller13/signal generator1/Drive_Signal3 ==
  QuasiEnable : Inport
  Frequency : Inport  Port=2
  Offset : Inport  Port=3
  Amplitude : Inport  Port=4
  PitchBias : Inport  Port=5
  split cycle mu : Inport  Port=6
  AveragedAmp_filtered : Subsystem  Commented=through
  AveragedOffset_filtered : Subsystem  Commented=through
  AveragedTau_filtered : Subsystem
  OutputWithRamping : Product  RndMeth=Zero
  PreGain : Constant
  PrescaledAmp : Product  RndMeth=Zero
  PrescaledOffset : Product  RndMeth=Zero
  ProductPhase : Product  RndMeth=Zero
  RampUpOrDown : DiscreteIntegrator  gainval=100  SampleTime=-1  LimitOutput=on  UpperSaturationLimit=1  LowerSaturationLimit=0  ICPrevOutput=DiscIntNeverNeededParam  ICPrevScaledInput=DiscIntNeverNeededParam
  SignalForRamp_binary : Subsystem
  SignalForSin_binary : Subsystem
  Subsystem : Subsystem
  Sum : Sum
  Sum1 : Sum
  signal with gain : Product  RndMeth=Zero
  SignalOutput : Outport
  WithoutRamp : Outport  Port=2
  RampOutput : Outport  Port=3
  AmplitudeOutput : Outport  Port=4
  OffsetOutput : Outport  Port=5
  wires:
  PrescaledAmp/1 -> AveragedAmp_filtered/1(In1)
  Sum/1 -> OutputWithRamping/2, WithoutRamp/1
  RampUpOrDown/1 -> RampOutput/1, OutputWithRamping/1, SignalForSin_binary/1(In1)
  QuasiEnable/1 -> SignalForRamp_binary/1(In1)
  SignalForRamp_binary/1(Out1) -> RampUpOrDown/1
  Amplitude/1 -> PrescaledAmp/1
  signal with gain/1 -> Sum/1
  Frequency/1 -> ProductPhase/2
  SignalForSin_binary/1(Out1) -> ProductPhase/1
  ProductPhase/1 -> Subsystem/2(In2)
  AveragedOffset_filtered/1(Out1) -> Sum/2, OffsetOutput/1
  PrescaledOffset/1 -> AveragedOffset_filtered/1(In1)
  PreGain/1 -> PrescaledAmp/2, PrescaledOffset/2
  OutputWithRamping/1 -> SignalOutput/1
  AveragedAmp_filtered/1(Out1) -> signal with gain/2, AmplitudeOutput/1
  Sum1/1 -> PrescaledOffset/1
  Offset/1 -> Sum1/1
  PitchBias/1 -> Sum1/2
  AveragedTau_filtered/1(Out1) -> Subsystem/1(split cycle mu)
  split cycle mu/1 -> AveragedTau_filtered/1(In1)
  Subsystem/1(split cycle signal) -> signal with gain/1

== system controller13/signal generator1/Drive_Signal4 ==
  QuasiEnable : Inport
  Frequency : Inport  Port=2
  Offset : Inport  Port=3
  Amplitude : Inport  Port=4
  PitchBias : Inport  Port=5
  split cycle mu : Inport  Port=6
  AveragedAmp_filtered : Subsystem
  AveragedOffset_filtered : Subsystem
  AveragedTau_filtered : Subsystem
  OutputWithRamping : Product  RndMeth=Zero
  PreGain : Constant
  PrescaledAmp : Product  RndMeth=Zero
  PrescaledOffset : Product  RndMeth=Zero
  ProductPhase : Product  RndMeth=Zero
  RampUpOrDown : DiscreteIntegrator  gainval=100  SampleTime=-1  LimitOutput=on  UpperSaturationLimit=1  LowerSaturationLimit=0  ICPrevOutput=DiscIntNeverNeededParam  ICPrevScaledInput=DiscIntNeverNeededParam
  SignalForRamp_binary : Subsystem
  SignalForSin_binary : Subsystem
  Subsystem : Subsystem
  Sum : Sum
  Sum1 : Sum
  signal with gain : Product  RndMeth=Zero
  SignalOutput : Outport
  WithoutRamp : Outport  Port=2
  RampOutput : Outport  Port=3
  AmplitudeOutput : Outport  Port=4
  OffsetOutput : Outport  Port=5
  wires:
  PrescaledAmp/1 -> AveragedAmp_filtered/1(In1)
  Sum/1 -> OutputWithRamping/2, WithoutRamp/1
  RampUpOrDown/1 -> RampOutput/1, OutputWithRamping/1, SignalForSin_binary/1(In1)
  QuasiEnable/1 -> SignalForRamp_binary/1(In1)
  SignalForRamp_binary/1(Out1) -> RampUpOrDown/1
  Amplitude/1 -> PrescaledAmp/1
  signal with gain/1 -> Sum/1
  Frequency/1 -> ProductPhase/2
  SignalForSin_binary/1(Out1) -> ProductPhase/1
  ProductPhase/1 -> Subsystem/2(In2)
  AveragedOffset_filtered/1(Out1) -> Sum/2, OffsetOutput/1
  PrescaledOffset/1 -> AveragedOffset_filtered/1(In1)
  PreGain/1 -> PrescaledAmp/2, PrescaledOffset/2
  OutputWithRamping/1 -> SignalOutput/1
  AveragedAmp_filtered/1(Out1) -> signal with gain/2, AmplitudeOutput/1
  Sum1/1 -> PrescaledOffset/1
  Offset/1 -> Sum1/1
  PitchBias/1 -> Sum1/2
  AveragedTau_filtered/1(Out1) -> Subsystem/1(split cycle mu)
  split cycle mu/1 -> AveragedTau_filtered/1(In1)
  Subsystem/1(split cycle signal) -> signal with gain/1

== system controller13/signal generator1/SignalSaturationLimit ==
  BiasMax : Inport
  SignalRaw : Inport  Port=2
  GainBias : Gain
  MaxOf : MinMax  Function=max  Inputs=2
  MinOf : MinMax  Inputs=2
  ground : Constant
  SignalSatd : Outport
  wires:
  BiasMax/1 -> GainBias/1
  SignalRaw/1 -> MinOf/2
  MinOf/1 -> MaxOf/1
  MaxOf/1 -> SignalSatd/1
  GainBias/1 -> MinOf/1
  ground/1 -> MaxOf/2

== system controller13/signal generator1/SignalSaturationLimit1 ==
  BiasMax : Inport
  SignalRaw : Inport  Port=2
  GainBias : Gain
  MaxOf : MinMax  Function=max  Inputs=2
  MinOf : MinMax  Inputs=2
  ground : Constant
  SignalSatd : Outport
  wires:
  BiasMax/1 -> GainBias/1
  SignalRaw/1 -> MinOf/2
  MinOf/1 -> MaxOf/1
  MaxOf/1 -> SignalSatd/1
  GainBias/1 -> MinOf/1
  ground/1 -> MaxOf/2

== system controller13/signal generator1/SignalSaturationLimit2 ==
  BiasMax : Inport
  SignalRaw : Inport  Port=2
  GainBias : Gain
  MaxOf : MinMax  Function=max  Inputs=2
  MinOf : MinMax  Inputs=2
  ground : Constant
  SignalSatd : Outport
  wires:
  BiasMax/1 -> GainBias/1
  SignalRaw/1 -> MinOf/2
  MinOf/1 -> MaxOf/1
  MaxOf/1 -> SignalSatd/1
  GainBias/1 -> MinOf/1
  ground/1 -> MaxOf/2

== system controller13/signal generator1/SignalSaturationLimit3 ==
  BiasMax : Inport
  SignalRaw : Inport  Port=2
  GainBias : Gain
  MaxOf : MinMax  Function=max  Inputs=2
  MinOf : MinMax  Inputs=2
  ground : Constant
  SignalSatd : Outport
  wires:
  BiasMax/1 -> GainBias/1
  SignalRaw/1 -> MinOf/2
  MinOf/1 -> MaxOf/1
  MaxOf/1 -> SignalSatd/1
  GainBias/1 -> MinOf/1
  ground/1 -> MaxOf/2

== system controller13/signal generator1/signal generator 1 ==
  quasi enable : Inport
  max voltage : Inport  Port=2
  frequency : Inport  Port=3
  half amplitude : Inport  Port=4
  2pi : Gain  Gain=2*pi
  Add1 : Sum
  Add2 : Sum
  Gain1 : Gain  Gain=-1
  OutputWithRamping : Product  RndMeth=Zero
  RampUpOrDown : DiscreteIntegrator  gainval=100  SampleTime=-1  LimitOutput=on  UpperSaturationLimit=1  LowerSaturationLimit=0  ICPrevOutput=DiscIntNeverNeededParam  ICPrevScaledInput=DiscIntNeverNeededParam
  Scope : Scope
  Scope1 : Scope
  Scope2 : Scope
  SignalForRamp_binary : Subsystem
  SignalSaturationLimit4 : Subsystem
  Zero-Order Hold : ZeroOrderHold  SampleTime=1/400
  deg to rad : Gain  Gain=pi/180
  first harmonic : Trigonometry  Operator=cos  OutputSignalType=real
  get max voltage : Subsystem
  omega*t : DiscreteIntegrator  SampleTime=-1  ICPrevOutput=DiscIntNeverNeededParam  ICPrevScaledInput=DiscIntNeverNeededParam
  phase offset : Constant  Value=0
  signal with gain1 : Product  RndMeth=Zero
  SignalSatd : Outport
  wires:
  first harmonic/1 -> Gain1/1
  Zero-Order Hold/1 -> Add2/2, signal with gain1/2
  RampUpOrDown/1 -> OutputWithRamping/1
  deg to rad/1 -> Add1/1
  Add1/1 -> first harmonic/1
  max voltage/1 -> get max voltage/2(max voltage)
  2pi/1 -> omega*t/1
  signal with gain1/1 -> Add2/1
  Add2/1 -> OutputWithRamping/2
  omega*t/1 -> Add1/2
  Gain1/1 -> signal with gain1/1
  quasi enable/1 -> Scope2/1, SignalForRamp_binary/1(EnableSignal), get max voltage/1(QuasiEnable)
  SignalForRamp_binary/1(Out1) -> RampUpOrDown/1
  phase offset/1 -> deg to rad/1
  OutputWithRamping/1 -> Scope/1, SignalSaturationLimit4/2(SignalRaw)
  get max voltage/1(max signa;) -> Scope1/1, SignalSaturationLimit4/1(Max)
  SignalSaturationLimit4/1(SignalSatd) -> SignalSatd/1
  half amplitude/1 -> Zero-Order Hold/1
  frequency/1 -> 2pi/1

== system controller13/signal generator1/signal generator 2 ==
  quasi enable : Inport
  max voltage : Inport  Port=2
  frequency : Inport  Port=3
  half amplitude : Inport  Port=4
  2pi : Gain  Gain=2*pi
  Add1 : Sum
  Add2 : Sum
  Gain1 : Gain  Gain=-1
  OutputWithRamping : Product  RndMeth=Zero
  RampUpOrDown : DiscreteIntegrator  gainval=100  SampleTime=-1  LimitOutput=on  UpperSaturationLimit=1  LowerSaturationLimit=0  ICPrevOutput=DiscIntNeverNeededParam  ICPrevScaledInput=DiscIntNeverNeededParam
  SignalForRamp_binary : Subsystem
  SignalSaturationLimit4 : Subsystem
  Zero-Order Hold : ZeroOrderHold  SampleTime=1/400
  deg to rad : Gain  Gain=pi/180
  first harmonic : Trigonometry  Operator=cos  OutputSignalType=real
  get max voltage : Subsystem
  omega*t : DiscreteIntegrator  SampleTime=-1  ICPrevOutput=DiscIntNeverNeededParam  ICPrevScaledInput=DiscIntNeverNeededParam
  phase offset : Constant  Value=0
  signal with gain1 : Product  RndMeth=Zero
  SignalSatd : Outport
  wires:
  first harmonic/1 -> Gain1/1
  Zero-Order Hold/1 -> Add2/2, signal with gain1/2
  RampUpOrDown/1 -> OutputWithRamping/1
  deg to rad/1 -> Add1/1
  Add1/1 -> first harmonic/1
  max voltage/1 -> get max voltage/2(max voltage)
  2pi/1 -> omega*t/1
  signal with gain1/1 -> Add2/1
  Add2/1 -> OutputWithRamping/2
  omega*t/1 -> Add1/2
  Gain1/1 -> signal with gain1/1
  quasi enable/1 -> SignalForRamp_binary/1(EnableSignal), get max voltage/1(QuasiEnable)
  SignalForRamp_binary/1(Out1) -> RampUpOrDown/1
  phase offset/1 -> deg to rad/1
  OutputWithRamping/1 -> SignalSaturationLimit4/2(SignalRaw)
  get max voltage/1(max signa;) -> SignalSaturationLimit4/1(Max)
  SignalSaturationLimit4/1(SignalSatd) -> SignalSatd/1
  half amplitude/1 -> Zero-Order Hold/1
  frequency/1 -> 2pi/1

== system controller13/signal generator1/signal generator 3 ==
  quasi enable : Inport
  max voltage : Inport  Port=2
  frequency : Inport  Port=3
  half amplitude : Inport  Port=4
  2pi : Gain  Gain=2*pi
  Add1 : Sum
  Add2 : Sum
  Gain1 : Gain  Gain=-1
  OutputWithRamping : Product  RndMeth=Zero
  RampUpOrDown : DiscreteIntegrator  gainval=100  SampleTime=-1  LimitOutput=on  UpperSaturationLimit=1  LowerSaturationLimit=0  ICPrevOutput=DiscIntNeverNeededParam  ICPrevScaledInput=DiscIntNeverNeededParam
  SignalForRamp_binary : Subsystem
  SignalSaturationLimit4 : Subsystem
  Zero-Order Hold : ZeroOrderHold  SampleTime=1/400
  deg to rad : Gain  Gain=pi/180
  first harmonic : Trigonometry  Operator=cos  OutputSignalType=real
  get max voltage : Subsystem
  omega*t : DiscreteIntegrator  SampleTime=-1  ICPrevOutput=DiscIntNeverNeededParam  ICPrevScaledInput=DiscIntNeverNeededParam
  phase offset : Constant  Value=0
  signal with gain1 : Product  RndMeth=Zero
  SignalSatd : Outport
  wires:
  first harmonic/1 -> Gain1/1
  Zero-Order Hold/1 -> Add2/2, signal with gain1/2
  RampUpOrDown/1 -> OutputWithRamping/1
  deg to rad/1 -> Add1/1
  Add1/1 -> first harmonic/1
  max voltage/1 -> get max voltage/2(max voltage)
  2pi/1 -> omega*t/1
  signal with gain1/1 -> Add2/1
  Add2/1 -> OutputWithRamping/2
  omega*t/1 -> Add1/2
  Gain1/1 -> signal with gain1/1
  quasi enable/1 -> SignalForRamp_binary/1(EnableSignal), get max voltage/1(QuasiEnable)
  SignalForRamp_binary/1(Out1) -> RampUpOrDown/1
  phase offset/1 -> deg to rad/1
  OutputWithRamping/1 -> SignalSaturationLimit4/2(SignalRaw)
  get max voltage/1(max signa;) -> SignalSaturationLimit4/1(Max)
  SignalSaturationLimit4/1(SignalSatd) -> SignalSatd/1
  half amplitude/1 -> Zero-Order Hold/1
  frequency/1 -> 2pi/1

== system controller13/signal generator1/signal generator 4 ==
  quasi enable : Inport
  max voltage : Inport  Port=2
  frequency : Inport  Port=3
  half amplitude : Inport  Port=4
  2pi : Gain  Gain=2*pi
  Add1 : Sum
  Add2 : Sum
  Gain1 : Gain  Gain=-1
  OutputWithRamping : Product  RndMeth=Zero
  RampUpOrDown : DiscreteIntegrator  gainval=100  SampleTime=-1  LimitOutput=on  UpperSaturationLimit=1  LowerSaturationLimit=0  ICPrevOutput=DiscIntNeverNeededParam  ICPrevScaledInput=DiscIntNeverNeededParam
  SignalForRamp_binary : Subsystem
  SignalSaturationLimit4 : Subsystem
  Zero-Order Hold : ZeroOrderHold  SampleTime=1/400
  deg to rad : Gain  Gain=pi/180
  first harmonic : Trigonometry  Operator=cos  OutputSignalType=real
  get max voltage : Subsystem
  omega*t : DiscreteIntegrator  SampleTime=-1  ICPrevOutput=DiscIntNeverNeededParam  ICPrevScaledInput=DiscIntNeverNeededParam
  phase offset : Constant  Value=0
  signal with gain1 : Product  RndMeth=Zero
  SignalSatd : Outport
  wires:
  first harmonic/1 -> Gain1/1
  Zero-Order Hold/1 -> Add2/2, signal with gain1/2
  RampUpOrDown/1 -> OutputWithRamping/1
  deg to rad/1 -> Add1/1
  Add1/1 -> first harmonic/1
  max voltage/1 -> get max voltage/2(max voltage)
  2pi/1 -> omega*t/1
  signal with gain1/1 -> Add2/1
  Add2/1 -> OutputWithRamping/2
  omega*t/1 -> Add1/2
  Gain1/1 -> signal with gain1/1
  quasi enable/1 -> SignalForRamp_binary/1(EnableSignal), get max voltage/1(QuasiEnable)
  SignalForRamp_binary/1(Out1) -> RampUpOrDown/1
  phase offset/1 -> deg to rad/1
  OutputWithRamping/1 -> SignalSaturationLimit4/2(SignalRaw)
  get max voltage/1(max signa;) -> SignalSaturationLimit4/1(Max)
  SignalSaturationLimit4/1(SignalSatd) -> SignalSatd/1
  half amplitude/1 -> Zero-Order Hold/1
  frequency/1 -> 2pi/1

== system controller13/Jumping Simulation/Subsystem1/Subsystem ==
  "p q r " : Inport  OutDataTypeStr=double
  landing trigger : Inport  Port=2  OutDataTypeStr=double
  euler_landing : Inport  Port=3  OutDataTypeStr=double
  Rotation Angles to Direction Cosine Matrix : sharedtransform/Rotation Angles to Direction Cosine Matrix  rotationOrder=ZYX  aMode=aMode
  Selector : Selector  InputPortWidth=3  IndexOptions=Index vector (dialog)  Indices=[3 2 1]  OutputSizes=1
  Selector1 : Selector  InputPortWidth=3  IndexOptions=Index vector (dialog)  Indices=[3 2 1]  OutputSizes=1
  phi theta psi : Integrator  ExternalReset=rising  InitialConditionSource=external  InitialCondition=[0,0,0]  WrapState=on
  phidot thetadot psidot : shared6dofsys/DCM & Euler Angles (Euler)/phidot thetadot psidot  SystemSampleTime=-1  VariantActivationTime=update diagram  Latency=0  AutoFrameSizeCalculation=off
  DCM1 : Outport  OutDataTypeStr=double  VectorParamsAs1DForOutWhenUnconnected=off
  wires:
  phidot thetadot psidot/1 -> phi theta psi/1
  Rotation Angles to Direction Cosine Matrix/1 -> DCM1/1
  Selector/1 -> Rotation Angles to Direction Cosine Matrix/1
  "p q r "/1 -> phidot thetadot psidot/1
  phi theta psi/1 -> Selector/1, phidot thetadot psidot/2
  landing trigger/1 -> phi theta psi/2
  euler_landing/1 -> Selector1/1
  Selector1/1 -> phi theta psi/3
